simulink model "xplane2matlab"  (R2016a)
settings: Solver=ode45  StartTime=0.0  StopTime=inf  RelTol=1e-3
undefined symbols (not defined in the file): Cphi, degtorad, Kp, Kphi, Kr, tau
libraries: xpcutilitieslib x2, xpcobsoletelib x2, instrumentlib x2, simulink x1
settings Model: Creator=IEE12  LastModifiedBy=Marcelo
settings DataIOCC: LimitDataPoints=on  SaveFormat=Array
settings DebuggingCC: UnderspecifiedInitializationDetection=Classic  MergeDetectMultiDrivingBlocksExec=none  SolverPrmCheckMsg=warning  StateNameClashWarn=warning
settings HardwareCC: ProdBitPerPointer=32  ProdLargestAtomicFloat=None  ProdIntDivRoundTo=Undefined  ProdEndianess=Unspecified  ProdWordSize=32  ProdHWDeviceType=32-bit Generic
settings ModelReferenceCC: PropagateSignalLabelsOutOfModel=off
settings ConfigComp: CovModelRefEnable=Off

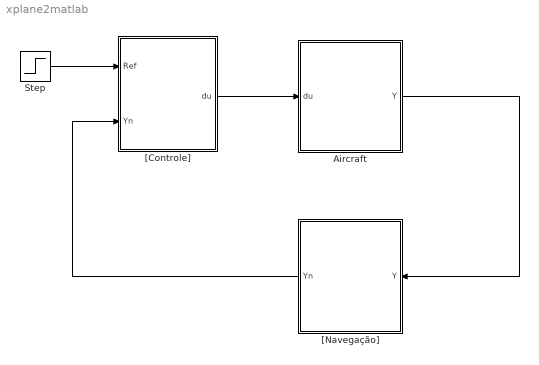
== system xplane2matlab ==
  Aircraft : Subsystem
  Step : Step  Time=0  After=degtorad(20)  SampleTime=0
  "[Controle]" : Subsystem
  "[Navegação]" : Subsystem
  wires:
  Step/1 -> "[Controle]"/1(Ref)
  "[Controle]"/1(du) -> Aircraft/1(du)
  Aircraft/1(Y) -> "[Navegação]"/1(Y)
  "[Navegação]"/1(Yn) -> "[Controle]"/2(Yn)

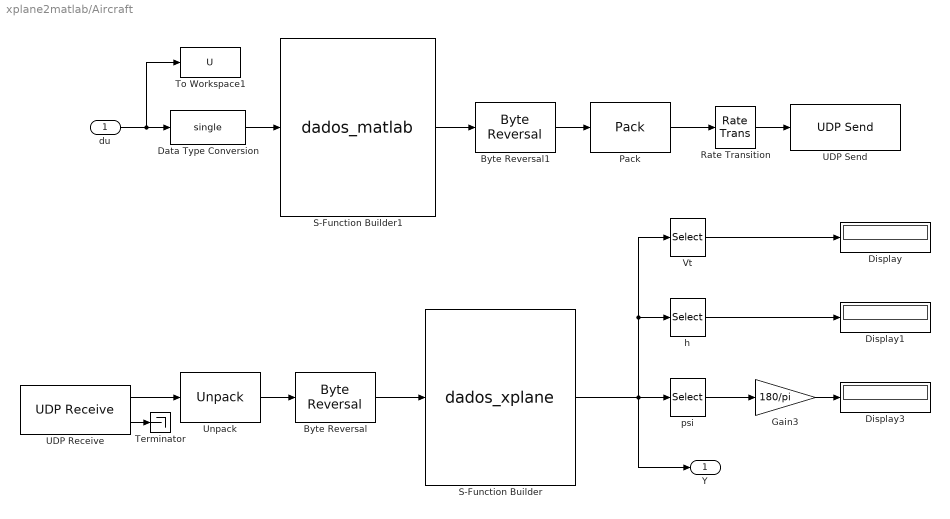
== system xplane2matlab/Aircraft ==
  du : Inport
  Byte Reversal : xpcutilitieslib/Byte Reversal   numInp=1
  Byte Reversal1 : xpcutilitieslib/Byte Reversal   numInp=1
  Data Type Conversion : DataTypeConversion  OutDataTypeStr=single
  Display : Display
  Display1 : Display
  Display3 : Display
  Gain3 : Gain  Gain=180/pi
  Pack : xpcobsoletelib/Utilities/Pack   datatypes={'uint8'}  byteAlign=1
  Rate Transition : RateTransition  OutPortSampleTime=0.02
  S-Function Builder : S-Function  InitFcn=try, set_param(gcb,'FunctionName','dados_xplane'), end  FunctionName=dados_xplane  SFunctionModules=dados_xplane_wrapper  SFunctionDeploymentMode=off  EnableBusSupport=off  mask(S-Function Builder){}
      mask help: Simulink:masks:SFunctionBuilder_MD
      mask init:
      | val = [[.9  0.75 0.75 1 1 .9 .9 1]',[1 1 0.75 0.75 .9 .9 1 .9]'];try , sys = get_param(gcb,'SfunBuilderFcnName');if isempty(sys), sys = get_param(gcb,'FunctionName'); end,catch, sys = get_param(gcb,'FunctionName'); end
      settings: CopyFcn=set_param(gcbh,'LinkStatus','none')  PreSaveFcn=try, set_param(gcb,'FunctionName','dados_xplane'), end  OpenFcn=sfunctionwizard(gcbh)
      mask Display: plot(val(:,1),val(:,2)),disp(sys), port_label('input',1,'Pkt'), port_label('output',1,'y')
  S-Function Builder1 : S-Function  InitFcn=try, set_param(gcb,'FunctionName','dados_matlab'), end  FunctionName=dados_matlab  SFunctionModules=dados_matlab_wrapper crc  SFunctionDeploymentMode=off  EnableBusSupport=off  mask(S-Function Builder){}
      mask help: Simulink:masks:SFunctionBuilder_MD
      mask init: same as xplane2matlab/Aircraft/S-Function Builder
      settings: CopyFcn=set_param(gcbh,'LinkStatus','none')  PreSaveFcn=try, set_param(gcb,'FunctionName','dados_matlab'), end  OpenFcn=sfunctionwizard(gcbh)
      mask Display: plot(val(:,1),val(:,2)),disp(sys), port_label('input',1,'u'), port_label('output',1,'Pkt')
  Terminator : Terminator
  To Workspace1 : ToWorkspace  VariableName=U  SaveFormat=Timeseries  SampleTime=-1
  UDP Receive : instrumentlib/UDP Receive  Host=127.0.0.1  Port=45004  LocalPort=45001  DataSize=77  EnableBlockingMode=off  Timeout=10  SampleTime=0.02  DataType=uint8  ByteOrder=BigEndian
  UDP Send : instrumentlib/UDP Send  Host=127.0.0.1  Port=45004  LocalPort=45001  EnableBlockingMode=on  ByteOrder=BigEndian
  Unpack : xpcobsoletelib/Utilities/Unpack   dimensions={[1 77]}  datatypes={'uint8'}  byteAlign=1
  Vt : Selector  InputPortWidth=12  IndexOptions=Index vector (dialog)  Indices=[1]  OutputSizes=1
  h : Selector  InputPortWidth=12  IndexOptions=Index vector (dialog)  Indices=[12]  OutputSizes=1
  psi : Selector  InputPortWidth=12  IndexOptions=Index vector (dialog)  Indices=[9]  OutputSizes=1
  Y : Outport
  wires:
  UDP Receive/2 -> Terminator/1
  UDP Receive/1 -> Unpack/1
  Unpack/1 -> Byte Reversal/1
  Byte Reversal/1 -> S-Function Builder/1
  Byte Reversal1/1 -> Pack/1
  S-Function Builder1/1 -> Byte Reversal1/1
  Pack/1 -> Rate Transition/1
  Data Type Conversion/1 -> S-Function Builder1/1
  psi/1 -> Gain3/1
  S-Function Builder/1 -> Y/1, Vt/1, h/1, psi/1
  Vt/1 -> Display/1
  h/1 -> Display1/1
  Gain3/1 -> Display3/1
  du/1 -> To Workspace1/1, Data Type Conversion/1
  Rate Transition/1 -> UDP Send/1

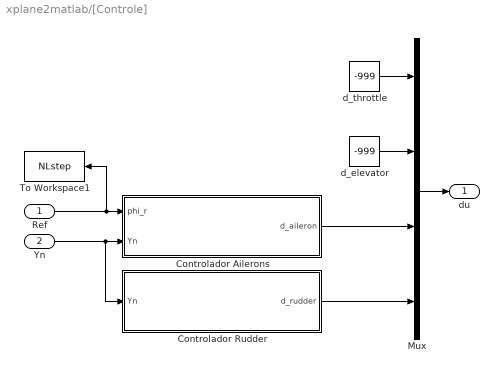
== system xplane2matlab/[Controle] ==
  Ref : Inport
  Yn : Inport  Port=2
  Controlador Ailerons : Subsystem
  Controlador Rudder : Subsystem
  Mux : Mux
  To Workspace1 : ToWorkspace  VariableName=NLstep  SaveFormat=Timeseries  SampleTime=-1
  d_elevator : Constant  Value=-999
  d_throttle : Constant  Value=-999
  du : Outport
  wires:
  Yn/1 -> Controlador Rudder/1(Yn), Controlador Ailerons/2(Yn)
  Mux/1 -> du/1
  Ref/1 -> To Workspace1/1, Controlador Ailerons/1(phi_r)
  Controlador Ailerons/1(d_aileron) -> Mux/3
  d_throttle/1 -> Mux/1
  d_elevator/1 -> Mux/2
  Controlador Rudder/1(d_rudder) -> Mux/4

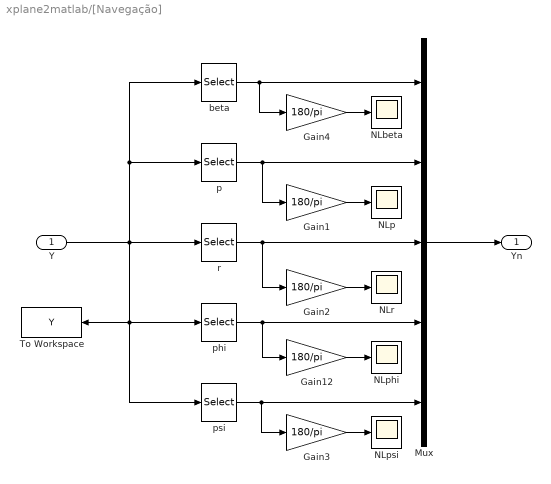
== system xplane2matlab/[Navegação] ==
  Y : Inport
  Gain{1..4,12} (5 alike) : Gain  Gain=180/pi
  Mux : Mux  Inputs=5
  NLbeta : Scope
  NLp : Scope
  NLphi : Scope
  NLpsi : Scope
  NLr : Scope
  To Workspace : ToWorkspace  VariableName=Y  SaveFormat=Timeseries  SampleTime=-1
  beta : Selector  InputPortWidth=12  IndexOptions=Index vector (dialog)  Indices=[3]  OutputSizes=1
  p : Selector  InputPortWidth=12  IndexOptions=Index vector (dialog)  Indices=[4]  OutputSizes=1
  phi : Selector  InputPortWidth=12  IndexOptions=Index vector (dialog)  Indices=[7]  OutputSizes=1
  psi : Selector  InputPortWidth=12  IndexOptions=Index vector (dialog)  Indices=[9]  OutputSizes=1
  r : Selector  InputPortWidth=12  IndexOptions=Index vector (dialog)  Indices=[6]  OutputSizes=1
  Yn : Outport
  wires:
  Y/1 -> phi/1, To Workspace/1, psi/1, beta/1, p/1, r/1
  Gain12/1 -> NLphi/1
  beta/1 -> Gain4/1, Mux/1
  phi/1 -> Gain12/1, Mux/4
  psi/1 -> Gain3/1, Mux/5
  Gain1/1 -> NLp/1
  p/1 -> Gain1/1, Mux/2
  Gain2/1 -> NLr/1
  r/1 -> Gain2/1, Mux/3
  Mux/1 -> Yn/1
  Gain3/1 -> NLpsi/1
  Gain4/1 -> NLbeta/1

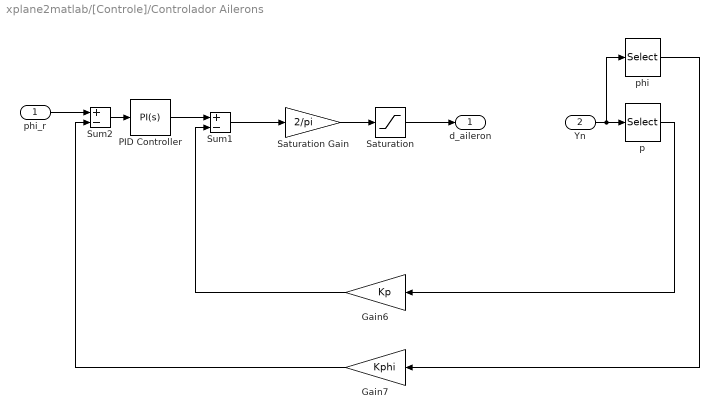
== system xplane2matlab/[Controle]/Controlador Ailerons ==
  phi_r : Inport
  Yn : Inport  Port=2
  Gain6 : Gain  Gain=Kp
  Gain7 : Gain  Gain=Kphi
  PID Controller : simulink/Continuous/PID Controller  Controller=PI  TimeDomain=Continuous-time  SampleTime=-1  IntegratorMethod=Forward Euler  FilterMethod=Forward Euler  Form=Parallel  UseFilter=on  ControllerParametersSource=internal  P=Cphi.Kp  I=Cphi.Ki  D=0  N=100  InitialConditionSource=internal  InitialConditionForIntegrator=0  InitialConditionForFilter=0  ExternalReset=none  ZeroCross=off  LimitOutput=off  UpperSaturationLimit=inf  LowerSaturationLimit=-inf  LinearizeAsGain=on  AntiWindupMode=none  Kb=1  TrackingMode=off  Kt=1  PParamMin=[]  PParamMax=[]  IParamMin=[]  IParamMax=[]  DParamMin=[]  DParamMax=[]  NParamMin=[]  NParamMax=[]  KbParamMin=[]  KbParamMax=[]  KtParamMin=[]  KtParamMax=[]  POutMin=[]  POutMax=[]  IOutMin=[]  IOutMax=[]  DOutMin=[]  DOutMax=[]  NOutMin=[]  NOutMax=[]  KbOutMin=[]  KbOutMax=[]  KtOutMin=[]  KtOutMax=[]  IntegratorOutMin=[]  IntegratorOutMax=[]  FilterOutMin=[]  FilterOutMax=[]  SumOutMin=[]  SumOutMax=[]  SumI1OutMin=[]  SumI1OutMax=[]  SumI2OutMin=[]  SumI2OutMax=[]  SumI3OutMin=[]  SumI3OutMax=[]  SumDOutMin=[]  SumDOutMax=[]  SaturationOutMin=[]  SaturationOutMax=[]  IntegratorContinuousStateAttributes=''  IntegratorStateMustResolveToSignalObject=off  IntegratorRTWStateStorageClass=Auto  FilterContinuousStateAttributes=''  FilterStateMustResolveToSignalObject=off  FilterRTWStateStorageClass=Auto  DifferentiatorICPrevScaledInput=0  DifferentiatorOutMin=[]  DifferentiatorOutMax=[]
  Saturation : Saturate
  Saturation Gain : Gain  Gain=2/pi
  Sum1 : Sum  Inputs=+-
  Sum2 : Sum  Inputs=+-
  p : Selector  InputPortWidth=5  IndexOptions=Index vector (dialog)  Indices=[2]  OutputSizes=1
  phi : Selector  InputPortWidth=5  IndexOptions=Index vector (dialog)  Indices=[4]  OutputSizes=1
  d_aileron : Outport
  wires:
  phi/1 -> Gain7/1
  p/1 -> Gain6/1
  Gain6/1 -> Sum1/2
  Gain7/1 -> Sum2/2
  PID Controller/1 -> Sum1/1
  Sum2/1 -> PID Controller/1
  Yn/1 -> phi/1, p/1
  phi_r/1 -> Sum2/1
  Saturation Gain/1 -> Saturation/1
  Saturation/1 -> d_aileron/1
  Sum1/1 -> Saturation Gain/1

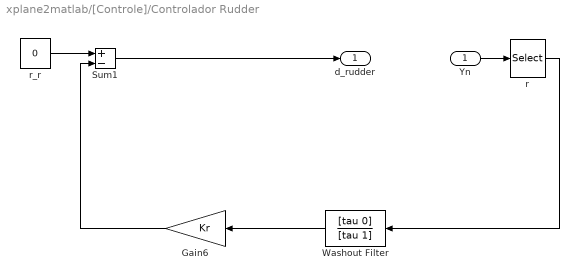
== system xplane2matlab/[Controle]/Controlador Rudder ==
  Yn : Inport
  Gain6 : Gain  Gain=Kr
  Sum1 : Sum  Inputs=+-
  Washout Filter : TransferFcn  Numerator=[tau 0]  Denominator=[tau 1]
  r : Selector  InputPortWidth=5  IndexOptions=Index vector (dialog)  Indices=[3]  OutputSizes=1
  r_r : Constant  Value=0
  d_rudder : Outport
  wires:
  r/1 -> Washout Filter/1
  Gain6/1 -> Sum1/2
  r_r/1 -> Sum1/1
  Yn/1 -> r/1
  Sum1/1 -> d_rudder/1
  Washout Filter/1 -> Gain6/1
